simulink model "hil_fuel_cell"  (R2023b)
settings: Solver=ode1  StartTime=0.0  StopTime=100  FixedStep=0.02  RelTol=1e-3  AbsTol=1e-3  EnableMultiTasking=on
model workspace: external: MATLAB File model_workspace.m (data not in the file)
CloseFcn:
  | try,close(h1_ssc_fuel_cell),end
  | clear h1_ssc_fuel_cell
  | try,close(h2_ssc_fuel_cell),end
  | clear h2_ssc_fuel_cell
  | try,close(h3_ssc_fuel_cell),end
  | clear h3_ssc_fuel_cell
  | try,close(h4_ssc_fuel_cell),end
  | clear h4_ssc_fuel_cell
  | try,close(h5_ssc_fuel_cell),end
  | clear h5_ssc_fuel_cell
  | 
  | clear tout simlog_ssc_fuel_cell
Description:
  | PEM Fuel Cell System
settings Model: Creator=The MathWorks, Inc.  LastModifiedBy=danie
settings ConfigSet: Description=VeriStand Targets (Windows & NI Linux Real-Time 64-bit)
settings SolverCC: AutoScaleAbsTol=off  MaxConsecutiveMinStep=2  AlgebraicLoopSolver=TrustRegion  AutoInsertRateTranBlk=on  InsertRTBMode=Always  MaxZcPerStep=1
settings OptimizationCC: DefaultParameterBehavior=Inlined  EnhancedBackFolding=on  PassReuseOutputArgsAs=Individual arguments  ZeroExternalMemoryAtStartup=off  ZeroInternalMemoryAtStartup=off  OptimizeBlockOrder=speed  DifferentSizesBufferReuse=on  OptimizationCustomize=off  EfficientTunableParamExpr=on
settings DebuggingCC: ParameterTunabilityLossMsg=error  UnconnectedInputMsg=warning  UnconnectedOutputMsg=warning  UnconnectedLineMsg=warning  SymbolicDimsDataTypeCodeGenerationDiagnostic=none
settings HardwareCC: ProdBitPerLong=64  ProdHWDeviceType=Intel->x86-64 (Linux 64)
settings ModelReferenceCC: EnableRefExpFcnMdlSchedulingChecks=on
settings SFSimCC: MATLABDynamicMemAlloc=off  CustomCodeUndefinedFunction=UseInterfaceOnly
settings RTWCC: Description=Embedded Coder  SystemTargetFile=ert.tlc  GenCodeOnly=on  PackageGeneratedCodeAndArtifacts=on  TemplateMakefile=ert_default_tmf  BuildConfiguration=Faster Runs  DLArmComputeVersion=19.05
settings CodeAppCC: ForceParamTrailComments=on  IgnoreCustomStorageClasses=off  OperatorAnnotations=on  SimulinkDataObjDesc=on  SFDataObjDesc=on  InsertBlockDesc=on
settings ERTTargetCC: TargetLangStandard=C99 (ISO)  GenerateSampleERTMain=on  SupportContinuousTime=on  InlinedParameterPlacement=NonHierarchical  ERTCustomFileTemplate=example_file_process.tlc
settings SimscapeCC: SimscapeLogName=simlog_ssc_fuel_cell  SimscapeLogDataHistory=20000

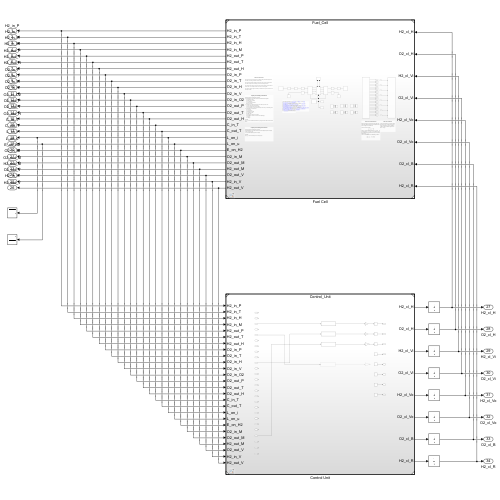
[thumbnail: Simulink's stored preview of the top-level diagram]
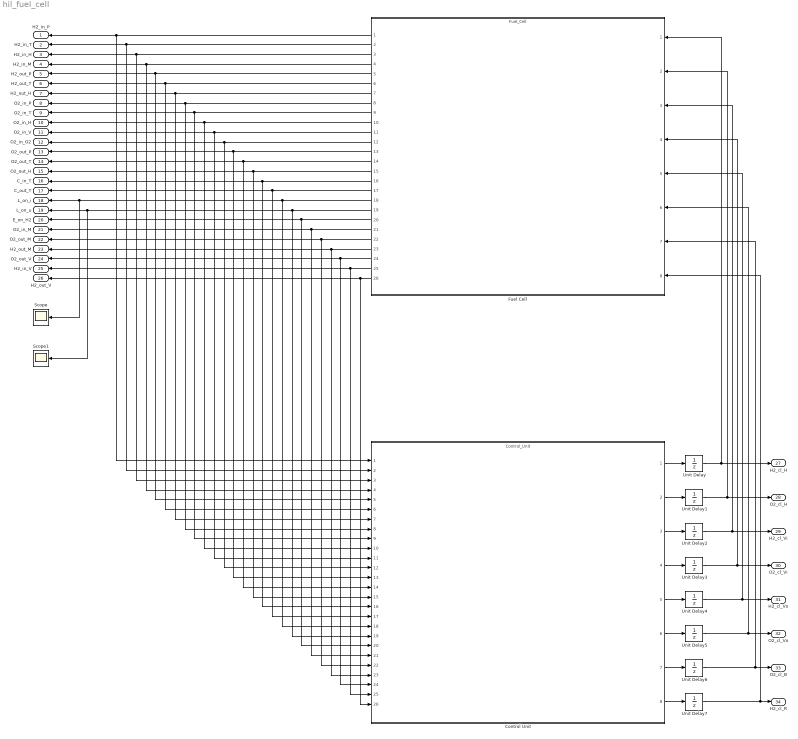
== system hil_fuel_cell ==
  Control Unit : ModelReference  ModelNameDialog=Control_Unit  SimulationMode=Normal  ModelReferenceVersion=5.4
  Fuel Cell : ModelReference  ModelNameDialog=Fuel_Cell  SimulationMode=Normal  ModelReferenceVersion=5.1
  Scope : Scope
  Scope1 : Scope
  Unit Delay{,1..7} (8 alike) : UnitDelay  SampleTime=-1  HasFrameUpgradeWarning=on
  H2_in_P : Outport
  H2_in_T : Outport  Port=2
  H2_in_H : Outport  Port=3
  H2_in_M : Outport  Port=4
  H2_out_P : Outport  Port=5
  H2_out_T : Outport  Port=6
  H2_out_H : Outport  Port=7
  O2_in_P : Outport  Port=8
  O2_in_T : Outport  Port=9
  O2_in_H : Outport  Port=10
  O2_in_V : Outport  Port=11
  O2_in_O2 : Outport  Port=12
  O2_out_P : Outport  Port=13
  O2_out_T : Outport  Port=14
  O2_out_H : Outport  Port=15
  C_in_T : Outport  Port=16
  C_out_T : Outport  Port=17
  L_on_i : Outport  Port=18
  L_on_u : Outport  Port=19
  E_on_H2 : Outport  Port=20
  O2_in_M : Outport  Port=21
  O2_out_M : Outport  Port=22
  H2_out_M : Outport  Port=23
  O2_out_V : Outport  Port=24
  H2_in_V : Outport  Port=25
  H2_out_V : Outport  Port=26
  H2_cl_H : Outport  Port=27
  O2_cl_H : Outport  Port=28
  H2_cl_Vi : Outport  Port=29
  O2_cl_Vi : Outport  Port=30
  H2_cl_Vo : Outport  Port=31
  O2_cl_Vo : Outport  Port=32
  O2_cl_B : Outport  Port=33
  H2_cl_R : Outport  Port=34
  wires:
  Control Unit/1 -> Unit Delay/1
  Control Unit/2 -> Unit Delay1/1
  Control Unit/3 -> Unit Delay2/1
  Control Unit/4 -> Unit Delay3/1
  Control Unit/5 -> Unit Delay4/1
  Fuel Cell/1 -> H2_in_P/1, Control Unit/1
  Fuel Cell/2 -> H2_in_T/1, Control Unit/2
  Fuel Cell/3 -> H2_in_H/1, Control Unit/3
  Fuel Cell/4 -> H2_in_M/1, Control Unit/4
  Fuel Cell/5 -> H2_out_P/1, Control Unit/5
  Fuel Cell/6 -> H2_out_T/1, Control Unit/6
  Fuel Cell/7 -> H2_out_H/1, Control Unit/7
  Fuel Cell/8 -> O2_in_P/1, Control Unit/8
  Fuel Cell/9 -> O2_in_T/1, Control Unit/9
  Fuel Cell/10 -> O2_in_H/1, Control Unit/10
  Fuel Cell/11 -> O2_in_V/1, Control Unit/11
  Fuel Cell/12 -> O2_in_O2/1, Control Unit/12
  Fuel Cell/13 -> O2_out_P/1, Control Unit/13
  Fuel Cell/14 -> O2_out_T/1, Control Unit/14
  Fuel Cell/15 -> O2_out_H/1, Control Unit/15
  Fuel Cell/16 -> C_in_T/1, Control Unit/16
  Fuel Cell/17 -> C_out_T/1, Control Unit/17
  Fuel Cell/18 -> Scope/1, L_on_i/1, Control Unit/18
  Fuel Cell/19 -> Scope1/1, L_on_u/1, Control Unit/19
  Fuel Cell/20 -> E_on_H2/1, Control Unit/20
  Fuel Cell/21 -> O2_in_M/1, Control Unit/21
  Fuel Cell/22 -> O2_out_M/1, Control Unit/22
  Fuel Cell/23 -> H2_out_M/1, Control Unit/23
  Fuel Cell/24 -> O2_out_V/1, Control Unit/24
  Fuel Cell/25 -> H2_in_V/1, Control Unit/25
  Fuel Cell/26 -> H2_out_V/1, Control Unit/26
  Control Unit/6 -> Unit Delay5/1
  Control Unit/7 -> Unit Delay6/1
  Control Unit/8 -> Unit Delay7/1
  Unit Delay/1 -> H2_cl_H/1, Fuel Cell/1
  Unit Delay1/1 -> O2_cl_H/1, Fuel Cell/2
  Unit Delay2/1 -> H2_cl_Vi/1, Fuel Cell/3
  Unit Delay3/1 -> O2_cl_Vi/1, Fuel Cell/4
  Unit Delay4/1 -> H2_cl_Vo/1, Fuel Cell/5
  Unit Delay5/1 -> Fuel Cell/6, O2_cl_Vo/1
  Unit Delay6/1 -> O2_cl_B/1, Fuel Cell/7
  Unit Delay7/1 -> H2_cl_R/1, Fuel Cell/8
